simulink model "Demo_16QAM"  (Simulink 6.0)
settings: Solver=ode45  StartTime=0.0  StopTime=200.0  RelTol=1e-3
libraries: commchan2 x1, commsink2 x1, commrandsrc2 x1, commdigbbndam2 x1
settings Model: LastModifiedBy=froze

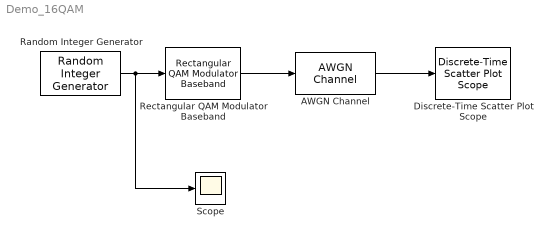
== system Demo_16QAM ==
  AWGN Channel : commchan2/AWGN Channel  seed=67  noiseMode="Signal to noise ratio  (Es/No)"  EbNodB=10  EsNodB=22  SNRdB=10  bitsPerSym=1  Ps=1  Tsym=0.1  variance=1
  Discrete-Time Scatter Plot Scope : commsink2/Discrete-Time Scatter Plot Scope  Tag=ScatterPlot  sampPerSymb=1  offsetEye=0  numTraces=4000  numNewFrames=1000  LineMarkers=.  LineColors=b  fading=on  render=on  AxisGrid=on  xMin=-1.5  xMax=1.5  yMin=-1.5  yMax=1.5  inphaseLabel=In-phase Amplitude  quadratureLabel=Quadrature Amplitude  openScopeAtSimStart=on  FrameNumber=off  FigPos=[360 60 560 560]  figTitle=Scatter Plot  numLinesMax=8  block_type_=scatter
  Random Integer Generator : commrandsrc2/Random Integer Generator  mul=16  seed=37  Ts=0.1  frameBased=off  sampPerFrame=1  orient=off
  Rectangular QAM Modulator Baseband : commdigbbndam2/Rectangular QAM Modulator Baseband  M=16  InType=Integer  Enc=Binary  PowType=Min. distance between symbols  MinDist=1  AvgPow=1  PeakPow=1  Ph=0  numSamp=4
  Scope : Scope
  wires:
  Random Integer Generator/1 -> Rectangular QAM Modulator Baseband/1, Scope/1
  Rectangular QAM Modulator Baseband/1 -> AWGN Channel/1
  AWGN Channel/1 -> Discrete-Time Scatter Plot Scope/1
